simulink model "gsm"  (R2015b)
settings: Solver=VariableStepDiscrete  StartTime=0.0  StopTime=inf  RelTol=1e-3
libraries: dspsigops x34, commblkintrlv2 x4, commdigbbndcpm2 x3, commcrc2 x2, commcnvcod2 x2, commsrccod2 x2, commrandsrc3 x1, commsink2 x1, commchan3 x1
(part 1 of 2)
settings Model: Creator=郭士坤  LastModifiedBy=郭士坤
settings DataIOCC: SaveFormat=Array  SignalLoggingSaveFormat=ModelDataLogs
settings OptimizationCC: InitFltsAndDblsToZero=on
settings DebuggingCC: SaveWithParameterizedLinksMsg=none  UnderspecifiedInitializationDetection=Classic  MergeDetectMultiDrivingBlocksExec=none  SignalResolutionControl=TryResolveAllWithWarning  SolverPrmCheckMsg=warning  MultiTaskDSMMsg=warning  MultiTaskCondExecSysMsg=none  FcnCallInpInsideContextMsg=EnableAllAsWarning
settings HardwareCC: ProdBitPerPointer=32  ProdLargestAtomicFloat=None  ProdIntDivRoundTo=Undefined  ProdEndianess=Unspecified  ProdWordSize=32  ProdHWDeviceType=32-bit Generic
settings SFSimCC: SimParseCustomCode=off
settings GRTTargetCC: TargetFcnLib=ansi_tfl_tmw.mat  CombineOutputUpdateFcns=off  GRTInterface=on
settings ConfigComp: CovModelRefEnable=Off
settings ConfigurationSet: Description=Simscape Multibody

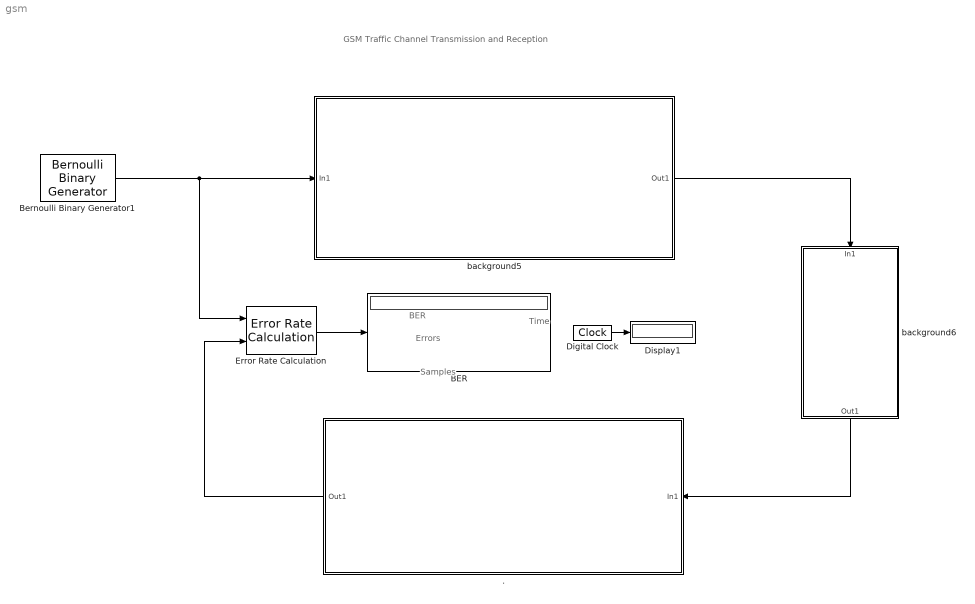
== system gsm ==
  note: GSM Traffic Channel
      | Transmission and
      | Reception
  note: Time
  note: BER
  note: Errors
  note: Samples
  . : Subsystem  Tag=Receiver
      mask Display: disp('Receiver')
  BER : Display
  Bernoulli Binary Generator1 : commrandsrc3/Bernoulli Binary Generator  ProbabilityOfZero=0.5  SeedSource=Auto  Seed=0  SampleTime=1/260  SamplesPerFrame=260  OutputDataType=double  SimulateUsing=Interpreted execution
  Digital Clock : DigitalClock  SampleTime=0.001
  Display1 : Display
  Error Rate Calculation : commsink2/Error Rate Calculation  N=520  st_delay=0  cp_mode=Entire frame  subframe=[]  PMode=Port  WsName=ErrorVec  RsMode2=off  stop=on  numErr=10000  maxBits=1e60
  background5 : Subsystem  Tag=Transmitter
      mask Display: disp('Transmitter')
  background6 : Subsystem
      mask Display: disp('Channel')
  wires:
  Error Rate Calculation/1 -> BER/1
  Digital Clock/1 -> Display1/1
  background5/1(Out1) -> background6/1(In1)
  ./1(Out1) -> Error Rate Calculation/2
  background6/1(Out1) -> ./1(In1)
  Bernoulli Binary Generator1/1 -> Error Rate Calculation/1, background5/1(In1)

== system gsm/. ==
  note: Receiver
  In1 : Inport
  Decoder : Subsystem
      mask Display: disp('Decoder')
  Demodulation : Subsystem
      mask Display: disp('Demodulation')
  Out1 : Outport
  wires:
  In1/1 -> Demodulation/1(In1)
  Demodulation/1(Out1) -> Decoder/1(In1)
  Decoder/1(Out1) -> Out1/1

== system gsm/background5 ==
  note: Transmitter
  In1 : Inport
  background2 : Subsystem
      mask Display: disp('Modulation')
  background5 : Subsystem  Tag=Codificación
      mask Display: disp('Coding')
  Out1 : Outport
  wires:
  background5/1(Out1) -> background2/1(In1)
  background2/1(Out1) -> Out1/1
  In1/1 -> background5/1(In1)

== system gsm/background6 ==
  note: Channel
  note: Raylenign fading Channel
  In1 : Inport
  GMSK Demodulator : commdigbbndcpm2/GMSK Demodulator Baseband  Commented=on  OutputType=Bit  BT=.3  pulseLength=1  preHistory=1  phaseOffset=0  samplesPerSymbol=1  RateOptions=Enforce single-rate processing  traceBack=1  outDType=double
  Multipath Rayleigh Fading Channel : commchan3/Multipath Rayleigh Fading Channel  maxDopplerShift=10  spectrumType=Jakes  sigmaGaussian=1/sqrt(2)  coeffRounded=[1 -1.72 0.785]  freqMinMaxRJakes=[0 1]  freqMinMaxAJakes=[0 1]  sigmaGaussian1=1/sqrt(2)  sigmaGaussian2=1/sqrt(2)  centerFreqGaussian1=0.0  centerFreqGaussian2=0.0  gainGaussian1=0.5  gainGaussian2=0.5  coeffBell=9  dopplerSpectrum=doppler.jakes  pathDelays=[0 2e-16]  avgPathGaindB=[0 -3]  normalizePathGains=on  seed=73  enableProbe=0  openVisAtStart=off  outPathGains=off  outDelay=off
  Out1 : Outport
  wires:
  In1/1 -> Multipath Rayleigh Fading Channel/1
  Multipath Rayleigh Fading Channel/1 -> Out1/1

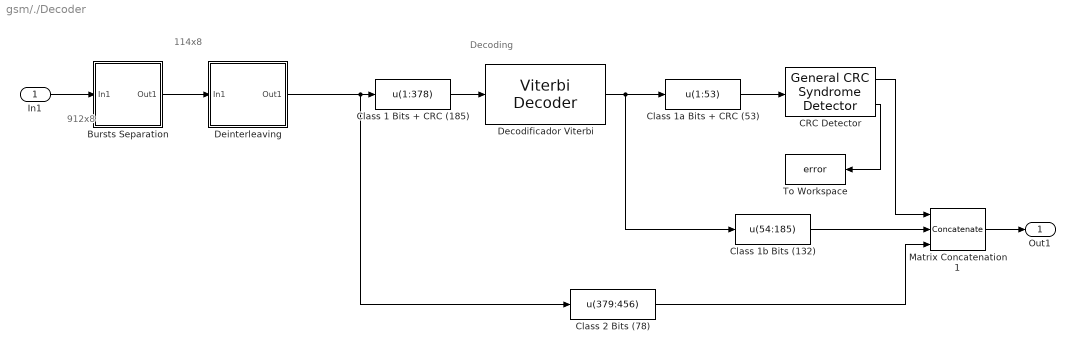
== system gsm/./Decoder ==
  note: 912x8
  note: 114x8
  note: Decoding
  In1 : Inport
  Bursts Separation : Subsystem
  CRC Detector : commcrc2/General CRC Syndrome Detector  genPoly=[1 1 0 1]  iniStates=[0]  directMethod=off  reflectInputBytes=off  reflectChecksums=off  finalXOR=0  numChecksums=1
  Class 1 Bits + CRC (185) : MATLABFcn  MATLABFcn=u(1:378)  OutputDimensions=[378,1]  Output1D=off
  Class 1a Bits + CRC (53) : MATLABFcn  MATLABFcn=u(1:53)  OutputDimensions=[53,1]  Output1D=off
  Class 1b Bits (132) : MATLABFcn  MATLABFcn=u(54:185)  OutputDimensions=[132,1]  Output1D=off
  Class 2 Bits (78) : MATLABFcn  MATLABFcn=u(379:456)  OutputDimensions=[78,1]  Output1D=off
  Decodificador Viterbi : commcnvcod2/Viterbi Decoder  trellis=poly2trellis(5, [31 33])  isPunctured=off  punctureVector=[1; 1; 0; 1; 0; 1]  erasures=off  dectype=Hard decision  nsdecb=4  runSigValErrCheck=off  tbdepth=10  opmode=Truncated  reset=off  delayedResetAction=off  smWordLength=16  outDataType=Inherit via internal rule
  Deinterleaving : Subsystem
  Matrix Concatenation1 : Concatenate  NumInputs=3  Mode=Multidimensional array
  To Workspace : ToWorkspace  VariableName=error  SampleTime=-1
  Out1 : Outport
  wires:
  Deinterleaving/1(Out1) -> Class 1 Bits + CRC (185)/1, Class 2 Bits (78)/1
  Class 1 Bits + CRC (185)/1 -> Decodificador Viterbi/1
  Decodificador Viterbi/1 -> Class 1a Bits + CRC (53)/1, Class 1b Bits (132)/1
  Class 1a Bits + CRC (53)/1 -> CRC Detector/1
  Class 2 Bits (78)/1 -> Matrix Concatenation1/3
  Class 1b Bits (132)/1 -> Matrix Concatenation1/2
  CRC Detector/1 -> Matrix Concatenation1/1
  CRC Detector/2 -> To Workspace/1
  Matrix Concatenation1/1 -> Out1/1
  Bursts Separation/1(Out1) -> Deinterleaving/1(In1)
  In1/1 -> Bursts Separation/1(In1)

== system gsm/./Demodulation ==
  note: Demodulation
  In1 : Inport
  Delay removal : MATLABFcn  MATLABFcn=u(17:1256+16)  OutputDimensions=[1256,1]  Output1D=off
  Differential Decoder : commsrccod2/Differential Decoder  InitCond=0
  GMSK Demodulator Baseband : commdigbbndcpm2/GMSK Demodulator Baseband  OutputType=Bit  BT=.3  pulseLength=1  preHistory=1  phaseOffset=0  samplesPerSymbol=1  RateOptions=Enforce single-rate processing  traceBack=16  outDType=double
  Reshape1 : Reshape  OutputDimensionality=Customize  OutputDimensions=[157,8]
  Out1 : Outport
  wires:
  Reshape1/1 -> Out1/1
  Differential Decoder/1 -> Reshape1/1
  GMSK Demodulator Baseband/1 -> Delay removal/1
  In1/1 -> GMSK Demodulator Baseband/1
  Delay removal/1 -> Differential Decoder/1

== system gsm/background5/background2 ==
  note: Modulation
  In1 : Inport
  Differential Encoder : commsrccod2/Differential Encoder  InitCond=0
  GMSK Modulator Baseband : commdigbbndcpm2/GMSK Modulator Baseband  inputType=Bit  BT=.3  pulseLength=1  preHistory=1  phaseOffset=0  samplesPerSymbol=1  RateOptions=Enforce single-rate processing  outDataType=double
  Reshape : Reshape  OutputDimensionality=Column vector (2-D)
  Zeros insertion : dspsigops/Pad  padAlong=Columns  dimsToPad=1  valSrc=Specify via dialog  padVal=0  spec=Output size  padNumOutRowsSpecMethod=User-specified  numOutRows=1256+16  padNumOutColsSpecMethod=User-specified  numOutCols=1  isVarDimsMode=off  padBeginning=0  padEnd=0  outSizeMode=User-specified  outSize=1  padSigAt=End  trunc_flag=None  roundingMode=Floor  overflowMode=off  truncOrWrapMode=Truncate  wrap_flag=None
  Out1 : Outport
  wires:
  In1/1 -> Reshape/1
  Reshape/1 -> Differential Encoder/1
  Differential Encoder/1 -> Zeros insertion/1
  GMSK Modulator Baseband/1 -> Out1/1
  Zeros insertion/1 -> GMSK Modulator Baseband/1

== system gsm/background5/background5 ==
  note: Coding
  In1 : Inport
  Calculation and adding of CRC : commcrc2/General CRC Generator  genPoly=[1 1 0 1]  iniStates=[0]  directMethod=off  reflectInputBytes=off  reflectChecksums=off  finalXOR=0  numChecksums=1
  Class 1a Bits (50) : MATLABFcn  MATLABFcn=u(1:50)  OutputDimensions=[50,1]  Output1D=off
  Class 1b Bits (132) : MATLABFcn  MATLABFcn=u(51:182)  OutputDimensions=[132,1]  Output1D=off
  Class 2 Bits (78) : MATLABFcn  MATLABFcn=u(183:260)  OutputDimensions=[78,1]  Output1D=off
  Convolutional Encoder : commcnvcod2/Convolutional Encoder  trellis=poly2trellis(5, [31 33])  opMode=Continuous  DelayedResetAction=off  hasIniStPort=off  hasFinStPort=off  usePuncVector=off  punctureVector=[1; 1; 0; 1; 0; 1]  reset=Unused parameter value
  Data Burst : Subsystem
  "Data Frame " : Concatenate  Mode=Multidimensional array
  Interleaving : Subsystem
  Matrix Assembler : Concatenate  Mode=Multidimensional array
  Zeros insertion : dspsigops/Pad  padAlong=Columns  dimsToPad=1  valSrc=Specify via dialog  padVal=0  spec=Output size  padNumOutRowsSpecMethod=User-specified  numOutRows=136  padNumOutColsSpecMethod=User-specified  numOutCols=1  isVarDimsMode=off  padBeginning=0  padEnd=0  outSizeMode=User-specified  outSize=1  padSigAt=End  trunc_flag=None  roundingMode=Floor  overflowMode=off  truncOrWrapMode=Truncate  wrap_flag=None
  Out1 : Outport
  wires:
  Class 1a Bits (50)/1 -> Calculation and adding of CRC/1
  Class 1b Bits (132)/1 -> Zeros insertion/1
  Matrix Assembler/1 -> Convolutional Encoder/1
  Convolutional Encoder/1 -> "Data Frame "/1
  Calculation and adding of CRC/1 -> Matrix Assembler/1
  Zeros insertion/1 -> Matrix Assembler/2
  Class 2 Bits (78)/1 -> "Data Frame "/2
  In1/1 -> Class 1a Bits (50)/1, Class 1b Bits (132)/1, Class 2 Bits (78)/1
  Interleaving/1("[114x8]") -> Data Burst/1(In1)
  Data Burst/1(Out1) -> Out1/1
  "Data Frame "/1 -> Interleaving/1("[912x1]")

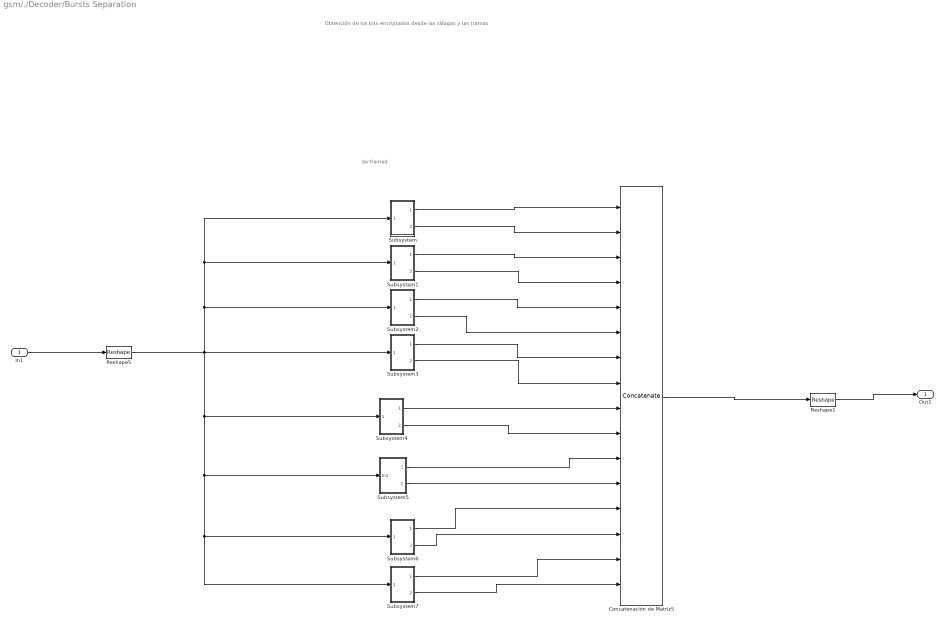
== system gsm/./Decoder/Bursts Separation ==
  note: de-framed
  note: Obtención de los bits encriptados
      | desde las ráfagas y las tramas
  In1 : Inport
  Concatenación de Matriz5 : Concatenate  NumInputs=16  Mode=Multidimensional array
  Reshape1 : Reshape  OutputDimensionality=Customize  OutputDimensions=[114,8]
  Reshape5 : Reshape  OutputDimensionality=Column vector (2-D)  OutputDimensions=[157,4]
  Subsystem : Subsystem
  Subsystem1 : Subsystem
  Subsystem2 : Subsystem
  Subsystem3 : Subsystem
  Subsystem4 : Subsystem
  Subsystem5 : Subsystem
  Subsystem6 : Subsystem
  Subsystem7 : Subsystem
  Out1 : Outport
  wires:
  In1/1 -> Reshape5/1
  Reshape5/1 -> Subsystem7/1(In1), Subsystem6/1(In1), Subsystem5/1(In1), Subsystem4/1(In1), Subsystem3/1(In1), Subsystem2/1(In1), Subsystem1/1(In1), Subsystem/1(In1)
  Reshape1/1 -> Out1/1
  Subsystem/1(Out1) -> Concatenación de Matriz5/1
  Subsystem/2(Out2) -> Concatenación de Matriz5/2
  Subsystem1/1(Out1) -> Concatenación de Matriz5/3
  Subsystem1/2(Out2) -> Concatenación de Matriz5/4
  Subsystem2/1(Out1) -> Concatenación de Matriz5/5
  Subsystem2/2(Out2) -> Concatenación de Matriz5/6
  Subsystem3/1(Out1) -> Concatenación de Matriz5/7
  Subsystem3/2(Out2) -> Concatenación de Matriz5/8
  Subsystem4/1(Out1) -> Concatenación de Matriz5/9
  Subsystem4/2(Out2) -> Concatenación de Matriz5/10
  Subsystem5/1(Out1) -> Concatenación de Matriz5/11
  Subsystem5/2(Out2) -> Concatenación de Matriz5/12
  Subsystem6/1(Out1) -> Concatenación de Matriz5/13
  Subsystem6/2(Out2) -> Concatenación de Matriz5/14
  Subsystem7/1(Out1) -> Concatenación de Matriz5/15
  Subsystem7/2(Out2) -> Concatenación de Matriz5/16
  Concatenación de Matriz5/1 -> Reshape1/1

== system gsm/./Decoder/Deinterleaving ==
  note: 可以往这里放一个enablesystem
  note: 第一次运行由于在Interlaveing中有一个912字节的buffer初始状态本来就有912个0，传出到了这里，所以s12中前面912是0
  note: Deinterleaving
  In1 : Inport
  Buffer : Buffer  N=456  TreatMby1Signals=One channel  OutputFrames=off
  Deinterleaver : commblkintrlv2/Matrix Deinterleaver  Nrows=114  Ncols=8
  Matrix Deinterleaver : commblkintrlv2/Matrix Deinterleaver  Nrows=57  Ncols=8
  Reshape : Reshape  OutputDimensionality=Column vector (2-D)
  Out1 : Outport
  wires:
  In1/1 -> Reshape/1
  Reshape/1 -> Deinterleaver/1
  Deinterleaver/1 -> Buffer/1
  Buffer/1 -> Matrix Deinterleaver/1
  Matrix Deinterleaver/1 -> Out1/1

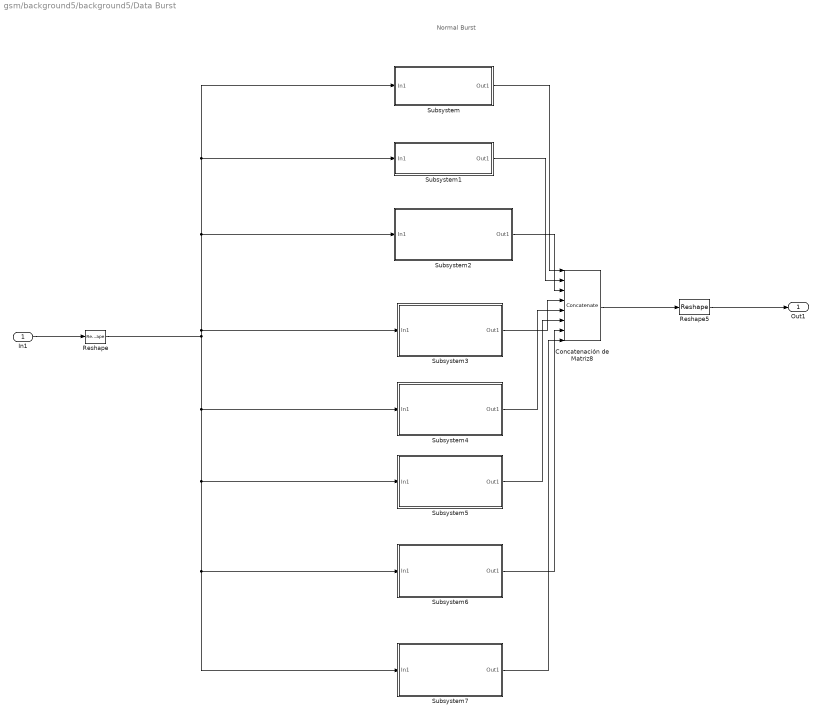
== system gsm/background5/background5/Data Burst ==
  note: Normal Burst
  In1 : Inport
  Concatenación de Matriz8 : Concatenate  NumInputs=8  Mode=Multidimensional array
  Reshape : Reshape  OutputDimensionality=Column vector (2-D)
  Reshape5 : Reshape  OutputDimensionality=Customize  OutputDimensions=[157,8]
  Subsystem : Subsystem
  Subsystem1 : Subsystem
  Subsystem2 : Subsystem
  Subsystem3 : Subsystem
  Subsystem4 : Subsystem
  Subsystem5 : Subsystem
  Subsystem6 : Subsystem
  Subsystem7 : Subsystem
  Out1 : Outport
  wires:
  In1/1 -> Reshape/1
  Concatenación de Matriz8/1 -> Reshape5/1
  Reshape5/1 -> Out1/1
  Subsystem/1(Out1) -> Concatenación de Matriz8/1
  Subsystem1/1(Out1) -> Concatenación de Matriz8/2
  Subsystem2/1(Out1) -> Concatenación de Matriz8/3
  Subsystem3/1(Out1) -> Concatenación de Matriz8/4
  Subsystem4/1(Out1) -> Concatenación de Matriz8/5
  Subsystem5/1(Out1) -> Concatenación de Matriz8/6
  Subsystem6/1(Out1) -> Concatenación de Matriz8/7
  Subsystem7/1(Out1) -> Concatenación de Matriz8/8
  Reshape/1 -> Subsystem3/1(In1), Subsystem/1(In1), Subsystem1/1(In1), Subsystem2/1(In1), Subsystem7/1(In1), Subsystem6/1(In1), Subsystem5/1(In1), Subsystem4/1(In1)

== system gsm/background5/background5/Interleaving ==
  note: Interleaving
  "[912x1]" : Inport
  Buffer : Buffer  N=912  TreatMby1Signals=One channel  OutputFrames=off
  Interleaver : commblkintrlv2/Matrix Interleaver  Nrows=57  Ncols=8
  Interleaver1 : commblkintrlv2/Matrix Interleaver  Nrows=114  Ncols=8
  Reshape : Reshape  OutputDimensionality=Customize  OutputDimensions=[114,8]
  To Workspace : ToWorkspace  VariableName=simout  SampleTime=-1
  "[114x8]" : Outport
  wires:
  "[912x1]"/1 -> Interleaver/1
  Interleaver/1 -> Buffer/1
  Buffer/1 -> To Workspace/1, Interleaver1/1
  Interleaver1/1 -> Reshape/1
  Reshape/1 -> "[114x8]"/1

== system gsm/./Decoder/Bursts Separation/Subsystem ==
  In1 : Inport
  Bits Encriptados  2 + SF2 : MATLABFcn  MATLABFcn=u(88:145)  OutputDimensions=[58,1]  Output1D=off
  Bits Encriptados 1 : MATLABFcn  MATLABFcn=u(4:60)  OutputDimensions=[57,1]  Output1D=off
  Bits Encriptados 1 + Tail Bits : MATLABFcn  MATLABFcn=u(1:60)  OutputDimensions=[60,1]  Output1D=off
  Bits Encriptados 1 + Tail Bits + SF1 : MATLABFcn  MATLABFcn=u(1:61)  OutputDimensions=[61,1]  Output1D=off
  Bits Encriptados 1 + Tail Bits + SF1 + Training : MATLABFcn  MATLABFcn=u(1:87)  OutputDimensions=[87,1]  Output1D=off
  Bits Encriptados 2 : MATLABFcn  MATLABFcn=u(2:58)  OutputDimensions=[57,1]  Output1D=off
  Trama 1 : MATLABFcn  MATLABFcn=u(1:157)  OutputDimensions=[157,1]  Output1D=off
  Trama1 - (Tail + Guard Bits) : MATLABFcn  MATLABFcn=u(1:145)  OutputDimensions=[145,1]  Output1D=off
  Out1 : Outport
  Out2 : Outport  Port=2
  wires:
  Bits Encriptados 1 + Tail Bits + SF1/1 -> Bits Encriptados 1 + Tail Bits/1
  Trama 1/1 -> Trama1 - (Tail + Guard Bits)/1
  Trama1 - (Tail + Guard Bits)/1 -> Bits Encriptados  2 + SF2/1, Bits Encriptados 1 + Tail Bits + SF1 + Training/1
  Bits Encriptados 1 + Tail Bits/1 -> Bits Encriptados 1/1
  Bits Encriptados 1 + Tail Bits + SF1 + Training/1 -> Bits Encriptados 1 + Tail Bits + SF1/1
  Bits Encriptados  2 + SF2/1 -> Bits Encriptados 2/1
  Bits Encriptados 1/1 -> Out1/1
  Bits Encriptados 2/1 -> Out2/1
  In1/1 -> Trama 1/1

== system gsm/./Decoder/Bursts Separation/Subsystem1 ==
  In1 : Inport
  Bits Encriptados  4 + SF2 : MATLABFcn  MATLABFcn=u(88:145)  OutputDimensions=[58,1]  Output1D=off
  Bits Encriptados 3 : MATLABFcn  MATLABFcn=u(4:60)  OutputDimensions=[57,1]  Output1D=off
  Bits Encriptados 3 + Tail Bits : MATLABFcn  MATLABFcn=u(1:60)  OutputDimensions=[60,1]  Output1D=off
  Bits Encriptados 3 + Tail Bits + SF1 : MATLABFcn  MATLABFcn=u(1:61)  OutputDimensions=[61,1]  Output1D=off
  Bits Encriptados 3 + Tail Bits + SF1 + Training1 : MATLABFcn  MATLABFcn=u(1:87)  OutputDimensions=[87,1]  Output1D=off
  Bits Encriptados 4 : MATLABFcn  MATLABFcn=u(2:58)  OutputDimensions=[57,1]  Output1D=off
  Trama 2 : MATLABFcn  MATLABFcn=u(158:314)  OutputDimensions=[157,1]  Output1D=off
  Trama2 - (Tail + Guard Bits) : MATLABFcn  MATLABFcn=u(1:145)  OutputDimensions=[145,1]  Output1D=off
  Out1 : Outport
  Out2 : Outport  Port=2
  wires:
  Bits Encriptados  4 + SF2/1 -> Bits Encriptados 4/1
  Bits Encriptados 3 + Tail Bits + SF1 + Training1/1 -> Bits Encriptados 3 + Tail Bits + SF1/1
  Bits Encriptados 3 + Tail Bits + SF1/1 -> Bits Encriptados 3 + Tail Bits/1
  Bits Encriptados 3 + Tail Bits/1 -> Bits Encriptados 3/1
  Trama2 - (Tail + Guard Bits)/1 -> Bits Encriptados  4 + SF2/1, Bits Encriptados 3 + Tail Bits + SF1 + Training1/1
  Trama 2/1 -> Trama2 - (Tail + Guard Bits)/1
  Bits Encriptados 3/1 -> Out1/1
  Bits Encriptados 4/1 -> Out2/1
  In1/1 -> Trama 2/1

== system gsm/./Decoder/Bursts Separation/Subsystem2 ==
  note: Bits Encriptados 7
      | + Tail Bits + SF1
  In1 : Inport
  Bits Encriptados  6 + SF2 : MATLABFcn  MATLABFcn=u(88:145)  OutputDimensions=[58,1]  Output1D=off
  Bits Encriptados 5 : MATLABFcn  MATLABFcn=u(4:60)  OutputDimensions=[57,1]  Output1D=off
  Bits Encriptados 5 + Tail Bits : MATLABFcn  MATLABFcn=u(1:60)  OutputDimensions=[60,1]  Output1D=off
  Bits Encriptados 5 + Tail Bits + SF1 : MATLABFcn  MATLABFcn=u(1:61)  OutputDimensions=[61,1]  Output1D=off
  Bits Encriptados 5 + Tail Bits + SF1 + Training2 : MATLABFcn  MATLABFcn=u(1:87)  OutputDimensions=[87,1]  Output1D=off
  Bits Encriptados 6 : MATLABFcn  MATLABFcn=u(2:58)  OutputDimensions=[57,1]  Output1D=off
  Trama 3 : MATLABFcn  MATLABFcn=u(315:471)  OutputDimensions=[157,1]  Output1D=off
  Trama3 - (Tail + Guard Bits) : MATLABFcn  MATLABFcn=u(1:145)  OutputDimensions=[145,1]  Output1D=off
  Out1 : Outport
  Out2 : Outport  Port=2
  wires:
  Trama 3/1 -> Trama3 - (Tail + Guard Bits)/1
  Bits Encriptados 5 + Tail Bits/1 -> Bits Encriptados 5/1
  Trama3 - (Tail + Guard Bits)/1 -> Bits Encriptados  6 + SF2/1, Bits Encriptados 5 + Tail Bits + SF1 + Training2/1
  Bits Encriptados 5 + Tail Bits + SF1 + Training2/1 -> Bits Encriptados 5 + Tail Bits + SF1/1
  Bits Encriptados 5 + Tail Bits + SF1/1 -> Bits Encriptados 5 + Tail Bits/1
  Bits Encriptados  6 + SF2/1 -> Bits Encriptados 6/1
  Bits Encriptados 5/1 -> Out1/1
  Bits Encriptados 6/1 -> Out2/1
  In1/1 -> Trama 3/1

== system gsm/./Decoder/Bursts Separation/Subsystem3 ==
  In1 : Inport
  Bits Encriptados  8 + SF2 : MATLABFcn  MATLABFcn=u(88:145)  OutputDimensions=[58,1]  Output1D=off
  Bits Encriptados 1 + Tail Bits + SF4 : MATLABFcn  MATLABFcn=u(1:61)  OutputDimensions=[61,1]  Output1D=off
  Bits Encriptados 7 : MATLABFcn  MATLABFcn=u(4:60)  OutputDimensions=[57,1]  Output1D=off
  Bits Encriptados 7 + Tail Bits : MATLABFcn  MATLABFcn=u(1:60)  OutputDimensions=[60,1]  Output1D=off
  Bits Encriptados 7 + Tail Bits + SF1 + Training : MATLABFcn  MATLABFcn=u(1:87)  OutputDimensions=[87,1]  Output1D=off
  Bits Encriptados 8 : MATLABFcn  MATLABFcn=u(2:58)  OutputDimensions=[57,1]  Output1D=off
  Trama 4 : MATLABFcn  MATLABFcn=u(472:628)  OutputDimensions=[157,1]  Output1D=off
  Trama4 - (Tail + Guard Bits) : MATLABFcn  MATLABFcn=u(1:145)  OutputDimensions=[145,1]  Output1D=off
  Out1 : Outport
  Out2 : Outport  Port=2
  wires:
  Bits Encriptados 7 + Tail Bits/1 -> Bits Encriptados 7/1
  Bits Encriptados  8 + SF2/1 -> Bits Encriptados 8/1
  Trama4 - (Tail + Guard Bits)/1 -> Bits Encriptados  8 + SF2/1, Bits Encriptados 7 + Tail Bits + SF1 + Training/1
  Trama 4/1 -> Trama4 - (Tail + Guard Bits)/1
  Bits Encriptados 7 + Tail Bits + SF1 + Training/1 -> Bits Encriptados 1 + Tail Bits + SF4/1
  Bits Encriptados 1 + Tail Bits + SF4/1 -> Bits Encriptados 7 + Tail Bits/1
  Bits Encriptados 7/1 -> Out1/1
  Bits Encriptados 8/1 -> Out2/1
  In1/1 -> Trama 4/1

== system gsm/./Decoder/Bursts Separation/Subsystem4 ==
  In1 : Inport
  Bits Encriptados  8 + SF2 : MATLABFcn  MATLABFcn=u(88:145)  OutputDimensions=[58,1]  Output1D=off
  Bits Encriptados 1 + Tail Bits + SF4 : MATLABFcn  MATLABFcn=u(1:61)  OutputDimensions=[61,1]  Output1D=off
  Bits Encriptados 7 : MATLABFcn  MATLABFcn=u(4:60)  OutputDimensions=[57,1]  Output1D=off
  Bits Encriptados 7 + Tail Bits : MATLABFcn  MATLABFcn=u(1:60)  OutputDimensions=[60,1]  Output1D=off
  Bits Encriptados 7 + Tail Bits + SF1 + Training : MATLABFcn  MATLABFcn=u(1:87)  OutputDimensions=[87,1]  Output1D=off
  Bits Encriptados 8 : MATLABFcn  MATLABFcn=u(2:58)  OutputDimensions=[57,1]  Output1D=off
  Trama 4 : MATLABFcn  MATLABFcn=u(629:785)  OutputDimensions=[157,1]  Output1D=off
  Trama4 - (Tail + Guard Bits) : MATLABFcn  MATLABFcn=u(1:145)  OutputDimensions=[145,1]  Output1D=off
  Out1 : Outport
  Out2 : Outport  Port=2
  wires:
  Bits Encriptados 7 + Tail Bits/1 -> Bits Encriptados 7/1
  Bits Encriptados  8 + SF2/1 -> Bits Encriptados 8/1
  Trama4 - (Tail + Guard Bits)/1 -> Bits Encriptados  8 + SF2/1, Bits Encriptados 7 + Tail Bits + SF1 + Training/1
  Trama 4/1 -> Trama4 - (Tail + Guard Bits)/1
  Bits Encriptados 7 + Tail Bits + SF1 + Training/1 -> Bits Encriptados 1 + Tail Bits + SF4/1
  Bits Encriptados 1 + Tail Bits + SF4/1 -> Bits Encriptados 7 + Tail Bits/1
  Bits Encriptados 7/1 -> Out1/1
  Bits Encriptados 8/1 -> Out2/1
  In1/1 -> Trama 4/1

== system gsm/./Decoder/Bursts Separation/Subsystem5 ==
  In1 : Inport
  Bits Encriptados  8 + SF2 : MATLABFcn  MATLABFcn=u(88:145)  OutputDimensions=[58,1]  Output1D=off
  Bits Encriptados 1 + Tail Bits + SF4 : MATLABFcn  MATLABFcn=u(1:61)  OutputDimensions=[61,1]  Output1D=off
  Bits Encriptados 7 : MATLABFcn  MATLABFcn=u(4:60)  OutputDimensions=[57,1]  Output1D=off
  Bits Encriptados 7 + Tail Bits : MATLABFcn  MATLABFcn=u(1:60)  OutputDimensions=[60,1]  Output1D=off
  Bits Encriptados 7 + Tail Bits + SF1 + Training : MATLABFcn  MATLABFcn=u(1:87)  OutputDimensions=[87,1]  Output1D=off
  Bits Encriptados 8 : MATLABFcn  MATLABFcn=u(2:58)  OutputDimensions=[57,1]  Output1D=off
  Trama 4 : MATLABFcn  MATLABFcn=u(786:942)  OutputDimensions=[157,1]  Output1D=off
  Trama4 - (Tail + Guard Bits) : MATLABFcn  MATLABFcn=u(1:145)  OutputDimensions=[145,1]  Output1D=off
  Out1 : Outport
  Out2 : Outport  Port=2
  wires:
  Bits Encriptados 7 + Tail Bits/1 -> Bits Encriptados 7/1
  Bits Encriptados  8 + SF2/1 -> Bits Encriptados 8/1
  Trama4 - (Tail + Guard Bits)/1 -> Bits Encriptados  8 + SF2/1, Bits Encriptados 7 + Tail Bits + SF1 + Training/1
  Trama 4/1 -> Trama4 - (Tail + Guard Bits)/1
  Bits Encriptados 7 + Tail Bits + SF1 + Training/1 -> Bits Encriptados 1 + Tail Bits + SF4/1
  Bits Encriptados 1 + Tail Bits + SF4/1 -> Bits Encriptados 7 + Tail Bits/1
  Bits Encriptados 7/1 -> Out1/1
  Bits Encriptados 8/1 -> Out2/1
  In1/1 -> Trama 4/1

== system gsm/./Decoder/Bursts Separation/Subsystem6 ==
  In1 : Inport
  Bits Encriptados  8 + SF2 : MATLABFcn  MATLABFcn=u(88:145)  OutputDimensions=[58,1]  Output1D=off
  Bits Encriptados 1 + Tail Bits + SF4 : MATLABFcn  MATLABFcn=u(1:61)  OutputDimensions=[61,1]  Output1D=off
  Bits Encriptados 7 : MATLABFcn  MATLABFcn=u(4:60)  OutputDimensions=[57,1]  Output1D=off
  Bits Encriptados 7 + Tail Bits : MATLABFcn  MATLABFcn=u(1:60)  OutputDimensions=[60,1]  Output1D=off
  Bits Encriptados 7 + Tail Bits + SF1 + Training : MATLABFcn  MATLABFcn=u(1:87)  OutputDimensions=[87,1]  Output1D=off
  Bits Encriptados 8 : MATLABFcn  MATLABFcn=u(2:58)  OutputDimensions=[57,1]  Output1D=off
  Trama 4 : MATLABFcn  MATLABFcn=u(943:1099)  OutputDimensions=[157,1]  Output1D=off
  Trama4 - (Tail + Guard Bits) : MATLABFcn  MATLABFcn=u(1:145)  OutputDimensions=[145,1]  Output1D=off
  Out1 : Outport
  Out2 : Outport  Port=2
  wires:
  Bits Encriptados 7 + Tail Bits/1 -> Bits Encriptados 7/1
  Bits Encriptados  8 + SF2/1 -> Bits Encriptados 8/1
  Trama4 - (Tail + Guard Bits)/1 -> Bits Encriptados  8 + SF2/1, Bits Encriptados 7 + Tail Bits + SF1 + Training/1
  Trama 4/1 -> Trama4 - (Tail + Guard Bits)/1
  Bits Encriptados 7 + Tail Bits + SF1 + Training/1 -> Bits Encriptados 1 + Tail Bits + SF4/1
  Bits Encriptados 1 + Tail Bits + SF4/1 -> Bits Encriptados 7 + Tail Bits/1
  Bits Encriptados 7/1 -> Out1/1
  Bits Encriptados 8/1 -> Out2/1
  In1/1 -> Trama 4/1

== system gsm/./Decoder/Bursts Separation/Subsystem7 ==
  In1 : Inport
  Bits Encriptados  8 + SF2 : MATLABFcn  MATLABFcn=u(88:145)  OutputDimensions=[58,1]  Output1D=off
  Bits Encriptados 1 + Tail Bits + SF4 : MATLABFcn  MATLABFcn=u(1:61)  OutputDimensions=[61,1]  Output1D=off
  Bits Encriptados 7 : MATLABFcn  MATLABFcn=u(4:60)  OutputDimensions=[57,1]  Output1D=off
  Bits Encriptados 7 + Tail Bits : MATLABFcn  MATLABFcn=u(1:60)  OutputDimensions=[60,1]  Output1D=off
  Bits Encriptados 7 + Tail Bits + SF1 + Training : MATLABFcn  MATLABFcn=u(1:87)  OutputDimensions=[87,1]  Output1D=off
  Bits Encriptados 8 : MATLABFcn  MATLABFcn=u(2:58)  OutputDimensions=[57,1]  Output1D=off
  Trama 4 : MATLABFcn  MATLABFcn=u(1100:1256)  OutputDimensions=[157,1]  Output1D=off
  Trama4 - (Tail + Guard Bits) : MATLABFcn  MATLABFcn=u(1:145)  OutputDimensions=[145,1]  Output1D=off
  Out1 : Outport
  Out2 : Outport  Port=2
  wires:
  Bits Encriptados 7 + Tail Bits/1 -> Bits Encriptados 7/1
  Bits Encriptados  8 + SF2/1 -> Bits Encriptados 8/1
  Trama4 - (Tail + Guard Bits)/1 -> Bits Encriptados  8 + SF2/1, Bits Encriptados 7 + Tail Bits + SF1 + Training/1
  Trama 4/1 -> Trama4 - (Tail + Guard Bits)/1
  Bits Encriptados 7 + Tail Bits + SF1 + Training/1 -> Bits Encriptados 1 + Tail Bits + SF4/1
  Bits Encriptados 1 + Tail Bits + SF4/1 -> Bits Encriptados 7 + Tail Bits/1
  Bits Encriptados 7/1 -> Out1/1
  Bits Encriptados 8/1 -> Out2/1
  In1/1 -> Trama 4/1

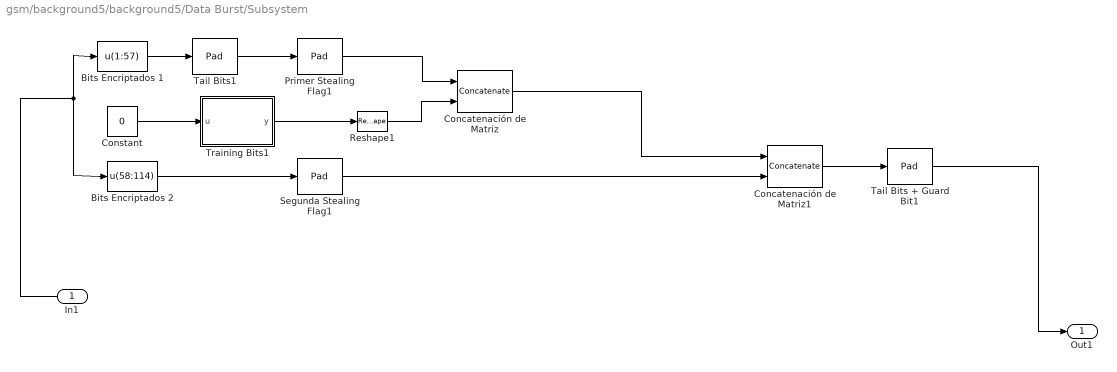
== system gsm/background5/background5/Data Burst/Subsystem ==
  In1 : Inport
  Bits Encriptados 1 : MATLABFcn  MATLABFcn=u(1:57)  OutputDimensions=[57,1]  Output1D=off
  Bits Encriptados 2 : MATLABFcn  MATLABFcn=u(58:114)  OutputDimensions=[57,1]  Output1D=off
  Concatenación de Matriz : Concatenate  Mode=Multidimensional array
  Concatenación de Matriz1 : Concatenate  Mode=Multidimensional array
  Constant : Constant  Value=0
  Primer Stealing Flag1 : dspsigops/Pad  padAlong=Columns  dimsToPad=1  valSrc=Specify via dialog  padVal=0  spec=Output size  padNumOutRowsSpecMethod=User-specified  numOutRows=61  padNumOutColsSpecMethod=User-specified  numOutCols=1  isVarDimsMode=off  padBeginning=0  padEnd=0  outSizeMode=User-specified  outSize=1  padSigAt=End  trunc_flag=None  roundingMode=Floor  overflowMode=off  truncOrWrapMode=Truncate  wrap_flag=None
  Reshape1 : Reshape  OutputDimensionality=Column vector (2-D)
  Segunda Stealing Flag1 : dspsigops/Pad  padAlong=Columns  dimsToPad=1  valSrc=Specify via dialog  padVal=0  spec=Output size  padNumOutRowsSpecMethod=User-specified  numOutRows=58  padNumOutColsSpecMethod=User-specified  numOutCols=1  isVarDimsMode=off  padBeginning=0  padEnd=0  outSizeMode=User-specified  outSize=1  padSigAt=Beginning  trunc_flag=None  roundingMode=Floor  overflowMode=off  truncOrWrapMode=Truncate  wrap_flag=None
  Tail Bits + Guard Bit1 : dspsigops/Pad  padAlong=Columns  dimsToPad=1  valSrc=Specify via dialog  padVal=0  spec=Output size  padNumOutRowsSpecMethod=User-specified  numOutRows=157  padNumOutColsSpecMethod=User-specified  numOutCols=1  isVarDimsMode=off  padBeginning=0  padEnd=0  outSizeMode=User-specified  outSize=1  padSigAt=End  trunc_flag=None  roundingMode=Floor  overflowMode=off  truncOrWrapMode=Truncate  wrap_flag=None
  Tail Bits1 : dspsigops/Pad  padAlong=Columns  dimsToPad=1  valSrc=Specify via dialog  padVal=0  spec=Output size  padNumOutRowsSpecMethod=User-specified  numOutRows=60  padNumOutColsSpecMethod=User-specified  numOutCols=1  isVarDimsMode=off  padBeginning=0  padEnd=0  outSizeMode=User-specified  outSize=1  padSigAt=Beginning  trunc_flag=None  roundingMode=Floor  overflowMode=off  truncOrWrapMode=Truncate  wrap_flag=None
  Training Bits1 : MATLAB Function  TreatAsAtomicUnit=on
      settings: PermitHierarchicalResolution=ParametersOnly
  Out1 : Outport
  wires:
  Tail Bits1/1 -> Primer Stealing Flag1/1
  Constant/1 -> Training Bits1/1(u)
  Concatenación de Matriz1/1 -> Tail Bits + Guard Bit1/1
  Concatenación de Matriz/1 -> Concatenación de Matriz1/1
  Reshape1/1 -> Concatenación de Matriz/2
  Bits Encriptados 2/1 -> Segunda Stealing Flag1/1
  Bits Encriptados 1/1 -> Tail Bits1/1
  Training Bits1/1(y) -> Reshape1/1
  Primer Stealing Flag1/1 -> Concatenación de Matriz/1
  Segunda Stealing Flag1/1 -> Concatenación de Matriz1/2
  Tail Bits + Guard Bit1/1 -> Out1/1
  In1/1 -> Bits Encriptados 1/1, Bits Encriptados 2/1

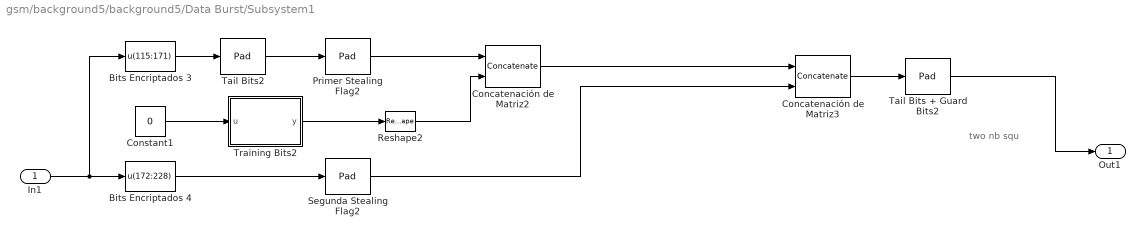
== system gsm/background5/background5/Data Burst/Subsystem1 ==
  note: two nb squ
  In1 : Inport
  Bits Encriptados 3 : MATLABFcn  MATLABFcn=u(115:171)  OutputDimensions=[57,1]  Output1D=off
  Bits Encriptados 4 : MATLABFcn  MATLABFcn=u(172:228)  OutputDimensions=[57,1]  Output1D=off
  Concatenación de Matriz2 : Concatenate  Mode=Multidimensional array
  Concatenación de Matriz3 : Concatenate  Mode=Multidimensional array
  Constant1 : Constant  Value=0
  Primer Stealing Flag2 : dspsigops/Pad  padAlong=Columns  dimsToPad=1  valSrc=Specify via dialog  padVal=0  spec=Output size  padNumOutRowsSpecMethod=User-specified  numOutRows=61  padNumOutColsSpecMethod=User-specified  numOutCols=1  isVarDimsMode=off  padBeginning=0  padEnd=0  outSizeMode=User-specified  outSize=1  padSigAt=End  trunc_flag=None  roundingMode=Floor  overflowMode=off  truncOrWrapMode=Truncate  wrap_flag=None
  Reshape2 : Reshape  OutputDimensionality=Column vector (2-D)
  Segunda Stealing Flag2 : dspsigops/Pad  padAlong=Columns  dimsToPad=1  valSrc=Specify via dialog  padVal=0  spec=Output size  padNumOutRowsSpecMethod=User-specified  numOutRows=58  padNumOutColsSpecMethod=User-specified  numOutCols=1  isVarDimsMode=off  padBeginning=0  padEnd=0  outSizeMode=User-specified  outSize=1  padSigAt=Beginning  trunc_flag=None  roundingMode=Floor  overflowMode=off  truncOrWrapMode=Truncate  wrap_flag=None
  Tail Bits + Guard Bits2 : dspsigops/Pad  padAlong=Columns  dimsToPad=1  valSrc=Specify via dialog  padVal=0  spec=Output size  padNumOutRowsSpecMethod=User-specified  numOutRows=157  padNumOutColsSpecMethod=User-specified  numOutCols=1  isVarDimsMode=off  padBeginning=0  padEnd=0  outSizeMode=User-specified  outSize=1  padSigAt=End  trunc_flag=None  roundingMode=Floor  overflowMode=off  truncOrWrapMode=Truncate  wrap_flag=None
  Tail Bits2 : dspsigops/Pad  padAlong=Columns  dimsToPad=1  valSrc=Specify via dialog  padVal=0  spec=Output size  padNumOutRowsSpecMethod=User-specified  numOutRows=60  padNumOutColsSpecMethod=User-specified  numOutCols=1  isVarDimsMode=off  padBeginning=0  padEnd=0  outSizeMode=User-specified  outSize=1  padSigAt=Beginning  trunc_flag=None  roundingMode=Floor  overflowMode=off  truncOrWrapMode=Truncate  wrap_flag=None
  Training Bits2 : MATLAB Function  TreatAsAtomicUnit=on
      settings: PermitHierarchicalResolution=ParametersOnly
  Out1 : Outport
  wires:
  Primer Stealing Flag2/1 -> Concatenación de Matriz2/1
  Constant1/1 -> Training Bits2/1(u)
  Concatenación de Matriz3/1 -> Tail Bits + Guard Bits2/1
  Reshape2/1 -> Concatenación de Matriz2/2
  Concatenación de Matriz2/1 -> Concatenación de Matriz3/1
  Segunda Stealing Flag2/1 -> Concatenación de Matriz3/2
  Tail Bits2/1 -> Primer Stealing Flag2/1
  Training Bits2/1(y) -> Reshape2/1
  Bits Encriptados 3/1 -> Tail Bits2/1
  Bits Encriptados 4/1 -> Segunda Stealing Flag2/1
  Tail Bits + Guard Bits2/1 -> Out1/1
  In1/1 -> Bits Encriptados 3/1, Bits Encriptados 4/1

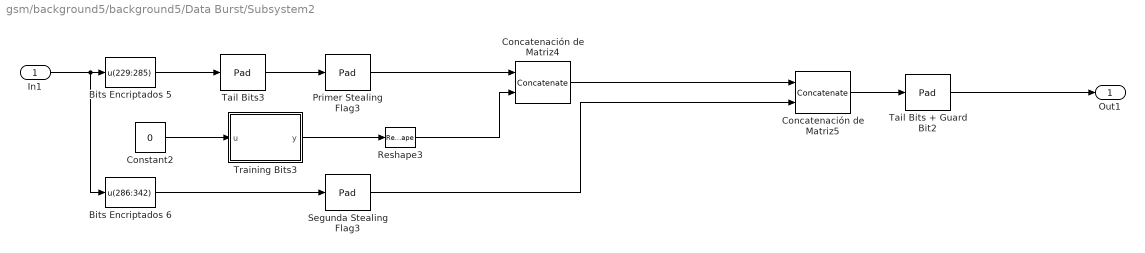
== system gsm/background5/background5/Data Burst/Subsystem2 ==
  In1 : Inport
  Bits Encriptados 5 : MATLABFcn  MATLABFcn=u(229:285)  OutputDimensions=[57,1]  Output1D=off
  Bits Encriptados 6 : MATLABFcn  MATLABFcn=u(286:342)  OutputDimensions=[57,1]  Output1D=off
  Concatenación de Matriz4 : Concatenate  Mode=Multidimensional array
  Concatenación de Matriz5 : Concatenate  Mode=Multidimensional array
  Constant2 : Constant  Value=0
  Primer Stealing Flag3 : dspsigops/Pad  padAlong=Columns  dimsToPad=1  valSrc=Specify via dialog  padVal=0  spec=Output size  padNumOutRowsSpecMethod=User-specified  numOutRows=61  padNumOutColsSpecMethod=User-specified  numOutCols=1  isVarDimsMode=off  padBeginning=0  padEnd=0  outSizeMode=User-specified  outSize=1  padSigAt=End  trunc_flag=None  roundingMode=Floor  overflowMode=off  truncOrWrapMode=Truncate  wrap_flag=None
  Reshape3 : Reshape  OutputDimensionality=Column vector (2-D)
  Segunda Stealing Flag3 : dspsigops/Pad  padAlong=Columns  dimsToPad=1  valSrc=Specify via dialog  padVal=0  spec=Output size  padNumOutRowsSpecMethod=User-specified  numOutRows=58  padNumOutColsSpecMethod=User-specified  numOutCols=1  isVarDimsMode=off  padBeginning=0  padEnd=0  outSizeMode=User-specified  outSize=1  padSigAt=Beginning  trunc_flag=None  roundingMode=Floor  overflowMode=off  truncOrWrapMode=Truncate  wrap_flag=None
  Tail Bits + Guard Bit2 : dspsigops/Pad  padAlong=Columns  dimsToPad=1  valSrc=Specify via dialog  padVal=0  spec=Output size  padNumOutRowsSpecMethod=User-specified  numOutRows=157  padNumOutColsSpecMethod=User-specified  numOutCols=1  isVarDimsMode=off  padBeginning=0  padEnd=0  outSizeMode=User-specified  outSize=1  padSigAt=End  trunc_flag=None  roundingMode=Floor  overflowMode=off  truncOrWrapMode=Truncate  wrap_flag=None
  Tail Bits3 : dspsigops/Pad  padAlong=Columns  dimsToPad=1  valSrc=Specify via dialog  padVal=0  spec=Output size  padNumOutRowsSpecMethod=User-specified  numOutRows=60  padNumOutColsSpecMethod=User-specified  numOutCols=1  isVarDimsMode=off  padBeginning=0  padEnd=0  outSizeMode=User-specified  outSize=1  padSigAt=Beginning  trunc_flag=None  roundingMode=Floor  overflowMode=off  truncOrWrapMode=Truncate  wrap_flag=None
  Training Bits3 : MATLAB Function  TreatAsAtomicUnit=on
      settings: PermitHierarchicalResolution=ParametersOnly
  Out1 : Outport
  wires:
  Training Bits3/1(y) -> Reshape3/1
  Reshape3/1 -> Concatenación de Matriz4/2
  Tail Bits3/1 -> Primer Stealing Flag3/1
  Bits Encriptados 5/1 -> Tail Bits3/1
  Bits Encriptados 6/1 -> Segunda Stealing Flag3/1
  Concatenación de Matriz4/1 -> Concatenación de Matriz5/1
  Constant2/1 -> Training Bits3/1(u)
  Tail Bits + Guard Bit2/1 -> Out1/1
  Concatenación de Matriz5/1 -> Tail Bits + Guard Bit2/1
  Primer Stealing Flag3/1 -> Concatenación de Matriz4/1
  Segunda Stealing Flag3/1 -> Concatenación de Matriz5/2
  In1/1 -> Bits Encriptados 6/1, Bits Encriptados 5/1

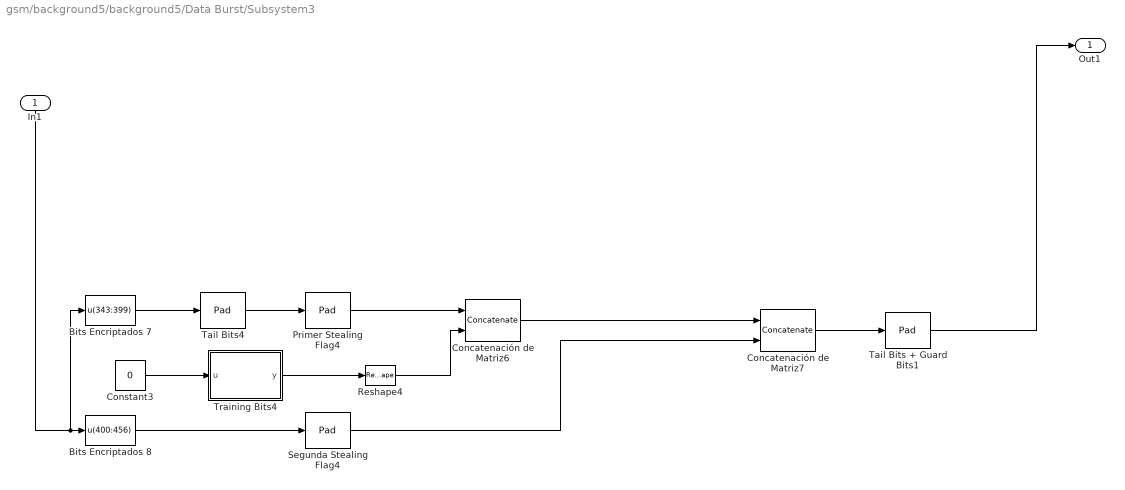
== system gsm/background5/background5/Data Burst/Subsystem3 ==
  In1 : Inport
  Bits Encriptados 7 : MATLABFcn  MATLABFcn=u(343:399)  OutputDimensions=[57,1]  Output1D=off
  Bits Encriptados 8 : MATLABFcn  MATLABFcn=u(400:456)  OutputDimensions=[57,1]  Output1D=off
  Concatenación de Matriz6 : Concatenate  Mode=Multidimensional array
  Concatenación de Matriz7 : Concatenate  Mode=Multidimensional array
  Constant3 : Constant  Value=0
  Primer Stealing Flag4 : dspsigops/Pad  padAlong=Columns  dimsToPad=1  valSrc=Specify via dialog  padVal=0  spec=Output size  padNumOutRowsSpecMethod=User-specified  numOutRows=61  padNumOutColsSpecMethod=User-specified  numOutCols=1  isVarDimsMode=off  padBeginning=0  padEnd=0  outSizeMode=User-specified  outSize=1  padSigAt=End  trunc_flag=None  roundingMode=Floor  overflowMode=off  truncOrWrapMode=Truncate  wrap_flag=None
  Reshape4 : Reshape  OutputDimensionality=Column vector (2-D)
  Segunda Stealing Flag4 : dspsigops/Pad  padAlong=Columns  dimsToPad=1  valSrc=Specify via dialog  padVal=0  spec=Output size  padNumOutRowsSpecMethod=User-specified  numOutRows=58  padNumOutColsSpecMethod=User-specified  numOutCols=1  isVarDimsMode=off  padBeginning=0  padEnd=0  outSizeMode=User-specified  outSize=1  padSigAt=Beginning  trunc_flag=None  roundingMode=Floor  overflowMode=off  truncOrWrapMode=Truncate  wrap_flag=None
  Tail Bits + Guard Bits1 : dspsigops/Pad  padAlong=Columns  dimsToPad=1  valSrc=Specify via dialog  padVal=0  spec=Output size  padNumOutRowsSpecMethod=User-specified  numOutRows=157  padNumOutColsSpecMethod=User-specified  numOutCols=1  isVarDimsMode=off  padBeginning=0  padEnd=0  outSizeMode=User-specified  outSize=1  padSigAt=End  trunc_flag=None  roundingMode=Floor  overflowMode=off  truncOrWrapMode=Truncate  wrap_flag=None
  Tail Bits4 : dspsigops/Pad  padAlong=Columns  dimsToPad=1  valSrc=Specify via dialog  padVal=0  spec=Output size  padNumOutRowsSpecMethod=User-specified  numOutRows=60  padNumOutColsSpecMethod=User-specified  numOutCols=1  isVarDimsMode=off  padBeginning=0  padEnd=0  outSizeMode=User-specified  outSize=1  padSigAt=Beginning  trunc_flag=None  roundingMode=Floor  overflowMode=off  truncOrWrapMode=Truncate  wrap_flag=None
  Training Bits4 : MATLAB Function  TreatAsAtomicUnit=on
      settings: PermitHierarchicalResolution=ParametersOnly
  Out1 : Outport
  wires:
  Training Bits4/1(y) -> Reshape4/1
  Tail Bits + Guard Bits1/1 -> Out1/1
  Concatenación de Matriz7/1 -> Tail Bits + Guard Bits1/1
  Primer Stealing Flag4/1 -> Concatenación de Matriz6/1
  Bits Encriptados 7/1 -> Tail Bits4/1
  Bits Encriptados 8/1 -> Segunda Stealing Flag4/1
  Tail Bits4/1 -> Primer Stealing Flag4/1
  Reshape4/1 -> Concatenación de Matriz6/2
  Segunda Stealing Flag4/1 -> Concatenación de Matriz7/2
  Constant3/1 -> Training Bits4/1(u)
  Concatenación de Matriz6/1 -> Concatenación de Matriz7/1
  In1/1 -> Bits Encriptados 8/1, Bits Encriptados 7/1

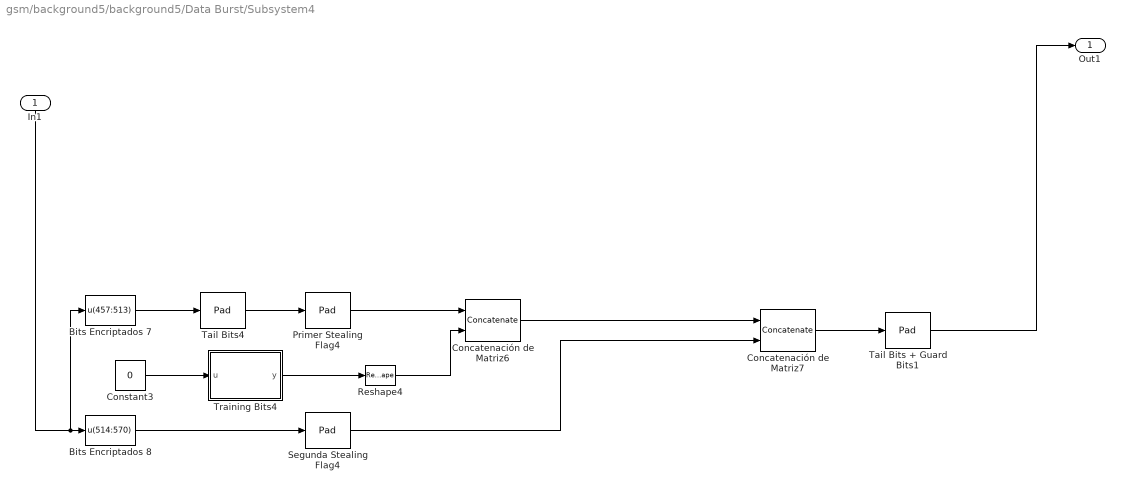
== system gsm/background5/background5/Data Burst/Subsystem4 ==
  In1 : Inport
  Bits Encriptados 7 : MATLABFcn  MATLABFcn=u(457:513)  OutputDimensions=[57,1]  Output1D=off
  Bits Encriptados 8 : MATLABFcn  MATLABFcn=u(514:570)  OutputDimensions=[57,1]  Output1D=off
  Concatenación de Matriz6 : Concatenate  Mode=Multidimensional array
  Concatenación de Matriz7 : Concatenate  Mode=Multidimensional array
  Constant3 : Constant  Value=0
  Primer Stealing Flag4 : dspsigops/Pad  padAlong=Columns  dimsToPad=1  valSrc=Specify via dialog  padVal=0  spec=Output size  padNumOutRowsSpecMethod=User-specified  numOutRows=61  padNumOutColsSpecMethod=User-specified  numOutCols=1  isVarDimsMode=off  padBeginning=0  padEnd=0  outSizeMode=User-specified  outSize=1  padSigAt=End  trunc_flag=None  roundingMode=Floor  overflowMode=off  truncOrWrapMode=Truncate  wrap_flag=None
  Reshape4 : Reshape  OutputDimensionality=Column vector (2-D)
  Segunda Stealing Flag4 : dspsigops/Pad  padAlong=Columns  dimsToPad=1  valSrc=Specify via dialog  padVal=0  spec=Output size  padNumOutRowsSpecMethod=User-specified  numOutRows=58  padNumOutColsSpecMethod=User-specified  numOutCols=1  isVarDimsMode=off  padBeginning=0  padEnd=0  outSizeMode=User-specified  outSize=1  padSigAt=Beginning  trunc_flag=None  roundingMode=Floor  overflowMode=off  truncOrWrapMode=Truncate  wrap_flag=None
  Tail Bits + Guard Bits1 : dspsigops/Pad  padAlong=Columns  dimsToPad=1  valSrc=Specify via dialog  padVal=0  spec=Output size  padNumOutRowsSpecMethod=User-specified  numOutRows=157  padNumOutColsSpecMethod=User-specified  numOutCols=1  isVarDimsMode=off  padBeginning=0  padEnd=0  outSizeMode=User-specified  outSize=1  padSigAt=End  trunc_flag=None  roundingMode=Floor  overflowMode=off  truncOrWrapMode=Truncate  wrap_flag=None
  Tail Bits4 : dspsigops/Pad  padAlong=Columns  dimsToPad=1  valSrc=Specify via dialog  padVal=0  spec=Output size  padNumOutRowsSpecMethod=User-specified  numOutRows=60  padNumOutColsSpecMethod=User-specified  numOutCols=1  isVarDimsMode=off  padBeginning=0  padEnd=0  outSizeMode=User-specified  outSize=1  padSigAt=Beginning  trunc_flag=None  roundingMode=Floor  overflowMode=off  truncOrWrapMode=Truncate  wrap_flag=None
  Training Bits4 : MATLAB Function  TreatAsAtomicUnit=on
      settings: PermitHierarchicalResolution=ParametersOnly
  Out1 : Outport
  wires:
  Training Bits4/1(y) -> Reshape4/1
  Tail Bits + Guard Bits1/1 -> Out1/1
  Concatenación de Matriz7/1 -> Tail Bits + Guard Bits1/1
  Primer Stealing Flag4/1 -> Concatenación de Matriz6/1
  Bits Encriptados 7/1 -> Tail Bits4/1
  Bits Encriptados 8/1 -> Segunda Stealing Flag4/1
  Tail Bits4/1 -> Primer Stealing Flag4/1
  Reshape4/1 -> Concatenación de Matriz6/2
  Segunda Stealing Flag4/1 -> Concatenación de Matriz7/2
  Constant3/1 -> Training Bits4/1(u)
  Concatenación de Matriz6/1 -> Concatenación de Matriz7/1
  In1/1 -> Bits Encriptados 8/1, Bits Encriptados 7/1

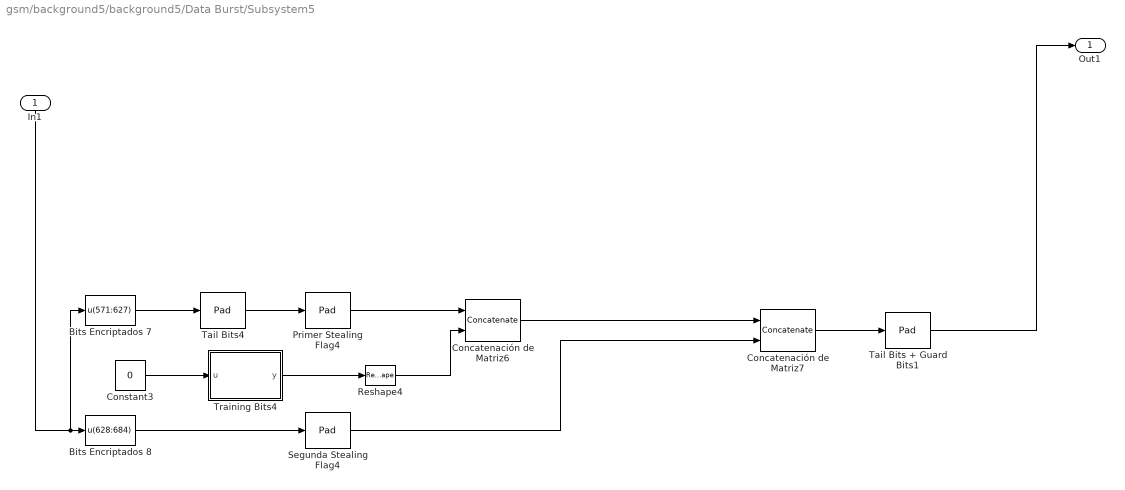
== system gsm/background5/background5/Data Burst/Subsystem5 ==
  In1 : Inport
  Bits Encriptados 7 : MATLABFcn  MATLABFcn=u(571:627)  OutputDimensions=[57,1]  Output1D=off
  Bits Encriptados 8 : MATLABFcn  MATLABFcn=u(628:684)  OutputDimensions=[57,1]  Output1D=off
  Concatenación de Matriz6 : Concatenate  Mode=Multidimensional array
  Concatenación de Matriz7 : Concatenate  Mode=Multidimensional array
  Constant3 : Constant  Value=0
  Primer Stealing Flag4 : dspsigops/Pad  padAlong=Columns  dimsToPad=1  valSrc=Specify via dialog  padVal=0  spec=Output size  padNumOutRowsSpecMethod=User-specified  numOutRows=61  padNumOutColsSpecMethod=User-specified  numOutCols=1  isVarDimsMode=off  padBeginning=0  padEnd=0  outSizeMode=User-specified  outSize=1  padSigAt=End  trunc_flag=None  roundingMode=Floor  overflowMode=off  truncOrWrapMode=Truncate  wrap_flag=None
  Reshape4 : Reshape  OutputDimensionality=Column vector (2-D)
  Segunda Stealing Flag4 : dspsigops/Pad  padAlong=Columns  dimsToPad=1  valSrc=Specify via dialog  padVal=0  spec=Output size  padNumOutRowsSpecMethod=User-specified  numOutRows=58  padNumOutColsSpecMethod=User-specified  numOutCols=1  isVarDimsMode=off  padBeginning=0  padEnd=0  outSizeMode=User-specified  outSize=1  padSigAt=Beginning  trunc_flag=None  roundingMode=Floor  overflowMode=off  truncOrWrapMode=Truncate  wrap_flag=None
  Tail Bits + Guard Bits1 : dspsigops/Pad  padAlong=Columns  dimsToPad=1  valSrc=Specify via dialog  padVal=0  spec=Output size  padNumOutRowsSpecMethod=User-specified  numOutRows=157  padNumOutColsSpecMethod=User-specified  numOutCols=1  isVarDimsMode=off  padBeginning=0  padEnd=0  outSizeMode=User-specified  outSize=1  padSigAt=End  trunc_flag=None  roundingMode=Floor  overflowMode=off  truncOrWrapMode=Truncate  wrap_flag=None
  Tail Bits4 : dspsigops/Pad  padAlong=Columns  dimsToPad=1  valSrc=Specify via dialog  padVal=0  spec=Output size  padNumOutRowsSpecMethod=User-specified  numOutRows=60  padNumOutColsSpecMethod=User-specified  numOutCols=1  isVarDimsMode=off  padBeginning=0  padEnd=0  outSizeMode=User-specified  outSize=1  padSigAt=Beginning  trunc_flag=None  roundingMode=Floor  overflowMode=off  truncOrWrapMode=Truncate  wrap_flag=None
  Training Bits4 : MATLAB Function  TreatAsAtomicUnit=on
      settings: PermitHierarchicalResolution=ParametersOnly
  Out1 : Outport
  wires:
  Training Bits4/1(y) -> Reshape4/1
  Tail Bits + Guard Bits1/1 -> Out1/1
  Concatenación de Matriz7/1 -> Tail Bits + Guard Bits1/1
  Primer Stealing Flag4/1 -> Concatenación de Matriz6/1
  Bits Encriptados 7/1 -> Tail Bits4/1
  Bits Encriptados 8/1 -> Segunda Stealing Flag4/1
  Tail Bits4/1 -> Primer Stealing Flag4/1
  Reshape4/1 -> Concatenación de Matriz6/2
  Segunda Stealing Flag4/1 -> Concatenación de Matriz7/2
  Constant3/1 -> Training Bits4/1(u)
  Concatenación de Matriz6/1 -> Concatenación de Matriz7/1
  In1/1 -> Bits Encriptados 8/1, Bits Encriptados 7/1

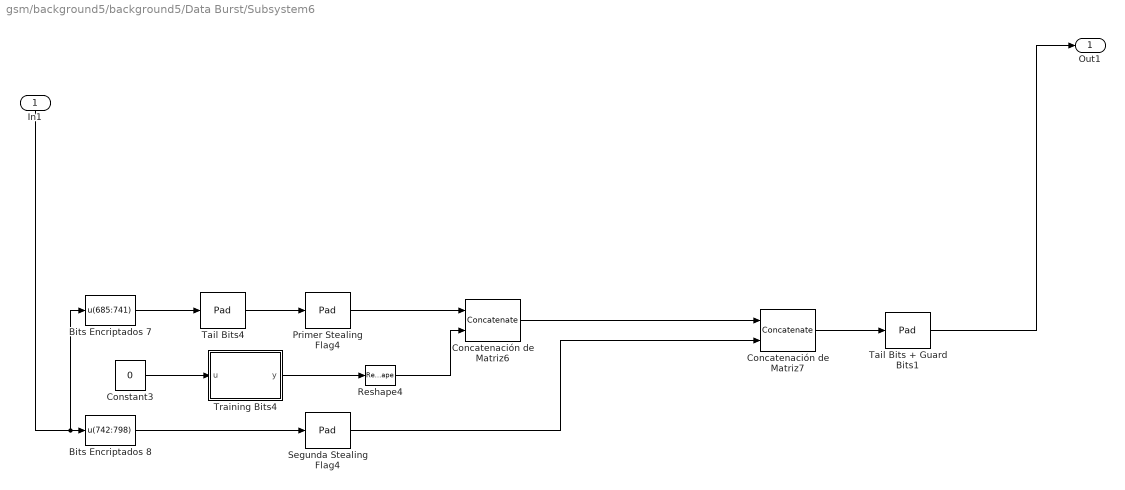
== system gsm/background5/background5/Data Burst/Subsystem6 ==
  In1 : Inport
  Bits Encriptados 7 : MATLABFcn  MATLABFcn=u(685:741)  OutputDimensions=[57,1]  Output1D=off
  Bits Encriptados 8 : MATLABFcn  MATLABFcn=u(742:798)  OutputDimensions=[57,1]  Output1D=off
  Concatenación de Matriz6 : Concatenate  Mode=Multidimensional array
  Concatenación de Matriz7 : Concatenate  Mode=Multidimensional array
  Constant3 : Constant  Value=0
  Primer Stealing Flag4 : dspsigops/Pad  padAlong=Columns  dimsToPad=1  valSrc=Specify via dialog  padVal=0  spec=Output size  padNumOutRowsSpecMethod=User-specified  numOutRows=61  padNumOutColsSpecMethod=User-specified  numOutCols=1  isVarDimsMode=off  padBeginning=0  padEnd=0  outSizeMode=User-specified  outSize=1  padSigAt=End  trunc_flag=None  roundingMode=Floor  overflowMode=off  truncOrWrapMode=Truncate  wrap_flag=None
  Reshape4 : Reshape  OutputDimensionality=Column vector (2-D)
  Segunda Stealing Flag4 : dspsigops/Pad  padAlong=Columns  dimsToPad=1  valSrc=Specify via dialog  padVal=0  spec=Output size  padNumOutRowsSpecMethod=User-specified  numOutRows=58  padNumOutColsSpecMethod=User-specified  numOutCols=1  isVarDimsMode=off  padBeginning=0  padEnd=0  outSizeMode=User-specified  outSize=1  padSigAt=Beginning  trunc_flag=None  roundingMode=Floor  overflowMode=off  truncOrWrapMode=Truncate  wrap_flag=None
  Tail Bits + Guard Bits1 : dspsigops/Pad  padAlong=Columns  dimsToPad=1  valSrc=Specify via dialog  padVal=0  spec=Output size  padNumOutRowsSpecMethod=User-specified  numOutRows=157  padNumOutColsSpecMethod=User-specified  numOutCols=1  isVarDimsMode=off  padBeginning=0  padEnd=0  outSizeMode=User-specified  outSize=1  padSigAt=End  trunc_flag=None  roundingMode=Floor  overflowMode=off  truncOrWrapMode=Truncate  wrap_flag=None
  Tail Bits4 : dspsigops/Pad  padAlong=Columns  dimsToPad=1  valSrc=Specify via dialog  padVal=0  spec=Output size  padNumOutRowsSpecMethod=User-specified  numOutRows=60  padNumOutColsSpecMethod=User-specified  numOutCols=1  isVarDimsMode=off  padBeginning=0  padEnd=0  outSizeMode=User-specified  outSize=1  padSigAt=Beginning  trunc_flag=None  roundingMode=Floor  overflowMode=off  truncOrWrapMode=Truncate  wrap_flag=None
  Training Bits4 : MATLAB Function  TreatAsAtomicUnit=on
      settings: PermitHierarchicalResolution=ParametersOnly
  Out1 : Outport
  wires:
  Training Bits4/1(y) -> Reshape4/1
  Tail Bits + Guard Bits1/1 -> Out1/1
  Concatenación de Matriz7/1 -> Tail Bits + Guard Bits1/1
  Primer Stealing Flag4/1 -> Concatenación de Matriz6/1
  Bits Encriptados 7/1 -> Tail Bits4/1
  Bits Encriptados 8/1 -> Segunda Stealing Flag4/1
  Tail Bits4/1 -> Primer Stealing Flag4/1
  Reshape4/1 -> Concatenación de Matriz6/2
  Segunda Stealing Flag4/1 -> Concatenación de Matriz7/2
  Constant3/1 -> Training Bits4/1(u)
  Concatenación de Matriz6/1 -> Concatenación de Matriz7/1
  In1/1 -> Bits Encriptados 8/1, Bits Encriptados 7/1

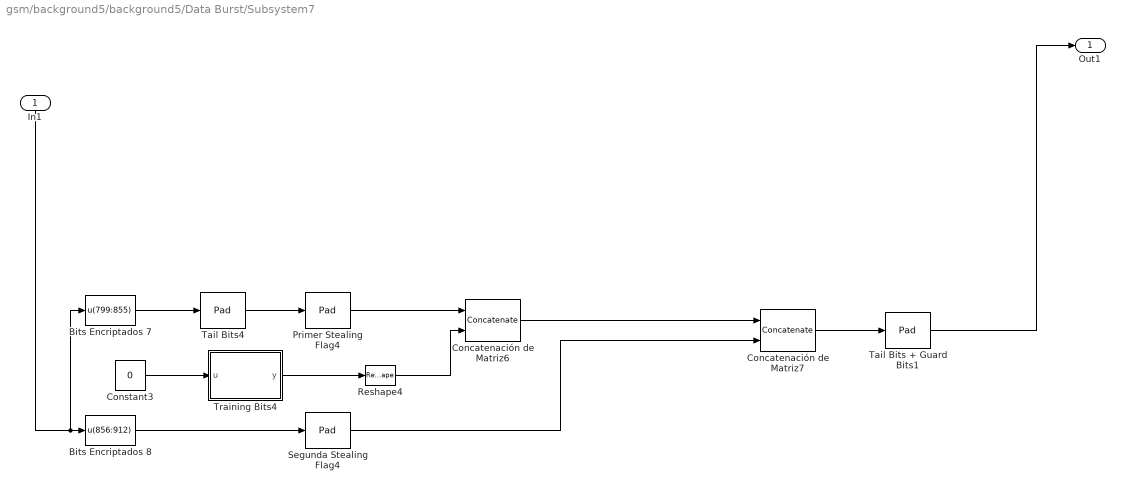
== system gsm/background5/background5/Data Burst/Subsystem7 ==
  In1 : Inport
  Bits Encriptados 7 : MATLABFcn  MATLABFcn=u(799:855)  OutputDimensions=[57,1]  Output1D=off
  Bits Encriptados 8 : MATLABFcn  MATLABFcn=u(856:912)  OutputDimensions=[57,1]  Output1D=off
  Concatenación de Matriz6 : Concatenate  Mode=Multidimensional array
  Concatenación de Matriz7 : Concatenate  Mode=Multidimensional array
  Constant3 : Constant  Value=0
  Primer Stealing Flag4 : dspsigops/Pad  padAlong=Columns  dimsToPad=1  valSrc=Specify via dialog  padVal=0  spec=Output size  padNumOutRowsSpecMethod=User-specified  numOutRows=61  padNumOutColsSpecMethod=User-specified  numOutCols=1  isVarDimsMode=off  padBeginning=0  padEnd=0  outSizeMode=User-specified  outSize=1  padSigAt=End  trunc_flag=None  roundingMode=Floor  overflowMode=off  truncOrWrapMode=Truncate  wrap_flag=None
  Reshape4 : Reshape  OutputDimensionality=Column vector (2-D)
  Segunda Stealing Flag4 : dspsigops/Pad  padAlong=Columns  dimsToPad=1  valSrc=Specify via dialog  padVal=0  spec=Output size  padNumOutRowsSpecMethod=User-specified  numOutRows=58  padNumOutColsSpecMethod=User-specified  numOutCols=1  isVarDimsMode=off  padBeginning=0  padEnd=0  outSizeMode=User-specified  outSize=1  padSigAt=Beginning  trunc_flag=None  roundingMode=Floor  overflowMode=off  truncOrWrapMode=Truncate  wrap_flag=None
  Tail Bits + Guard Bits1 : dspsigops/Pad  padAlong=Columns  dimsToPad=1  valSrc=Specify via dialog  padVal=0  spec=Output size  padNumOutRowsSpecMethod=User-specified  numOutRows=157  padNumOutColsSpecMethod=User-specified  numOutCols=1  isVarDimsMode=off  padBeginning=0  padEnd=0  outSizeMode=User-specified  outSize=1  padSigAt=End  trunc_flag=None  roundingMode=Floor  overflowMode=off  truncOrWrapMode=Truncate  wrap_flag=None
  Tail Bits4 : dspsigops/Pad  padAlong=Columns  dimsToPad=1  valSrc=Specify via dialog  padVal=0  spec=Output size  padNumOutRowsSpecMethod=User-specified  numOutRows=60  padNumOutColsSpecMethod=User-specified  numOutCols=1  isVarDimsMode=off  padBeginning=0  padEnd=0  outSizeMode=User-specified  outSize=1  padSigAt=Beginning  trunc_flag=None  roundingMode=Floor  overflowMode=off  truncOrWrapMode=Truncate  wrap_flag=None
  Training Bits4 : MATLAB Function  TreatAsAtomicUnit=on
      settings: PermitHierarchicalResolution=ParametersOnly
  Out1 : Outport
  wires:
  Training Bits4/1(y) -> Reshape4/1
  Tail Bits + Guard Bits1/1 -> Out1/1
  Concatenación de Matriz7/1 -> Tail Bits + Guard Bits1/1
  Primer Stealing Flag4/1 -> Concatenación de Matriz6/1
  Bits Encriptados 7/1 -> Tail Bits4/1
  Bits Encriptados 8/1 -> Segunda Stealing Flag4/1
  Tail Bits4/1 -> Primer Stealing Flag4/1
  Reshape4/1 -> Concatenación de Matriz6/2
  Segunda Stealing Flag4/1 -> Concatenación de Matriz7/2
  Constant3/1 -> Training Bits4/1(u)
  Concatenación de Matriz6/1 -> Concatenación de Matriz7/1
  In1/1 -> Bits Encriptados 8/1, Bits Encriptados 7/1

== matlab function gsm/background5/background5/Data Burst/Subsystem1/Training Bits2 ==
  data: u input; y output
function y = fcn(u)
% This block supports an embeddable subset of the MATLAB language.
% See the help menu for details. 

training2 = [0,0,1,0,1,1,0,1,1,1,0,1,1,1,1,0,0,0,1,0,1,1,0,1,1,1];
y = training2;

== matlab function gsm/background5/background5/Data Burst/Subsystem/Training Bits1 ==
  data: u input; y output
function y = fcn(u)
% This block supports an embeddable subset of the MATLAB language.
% See the help menu for details. 

training1 = [0,0,1,0,0,1,0,1,1,1,0,0,0,0,1,0,0,0,1,0,0,1,0,1,1,1];
y = training1;

== matlab function gsm/background5/background5/Data Burst/Subsystem2/Training Bits3 ==
  data: u input; y output
function y = fcn(u)
% This block supports an embeddable subset of the MATLAB language.
% See the help menu for details. 

training3 = [0,1,0,0,0,0,1,1,1,0,1,1,1,0,1,0,0,1,0,0,0,0,1,1,1,0];
y = training3;
